simulink model "img2017"  (R2016b)
settings: Solver=VariableStepAuto  StartTime=0.0  StopTime=40  RelTol=1e-3
undefined symbols (not defined in the file or in its folder): none, Rec, SDTV, videoinput
libraries: visionanalysis x2, visiontransforms x2, dspmtrx3 x2, visionconversions x1, visiontextngfix x1, visionstatistics x1, imaqlib x1, visionsinks x1
settings Model: Creator=Anushri-MacBook  LastModifiedBy=Anushri-MacBook

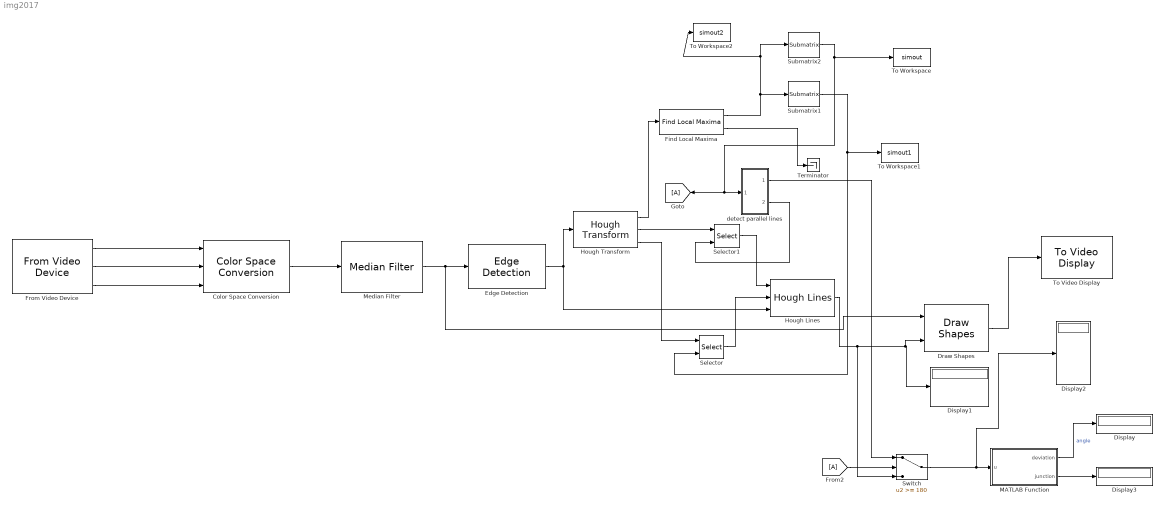
== system img2017 ==
  Color Space Conversion : visionconversions/Color Space  Conversion  conversion=Obsolete  conversionActive=R'G'B' to intensity  wp_str=D65  rec=Rec. 601 (SDTV)  sys=1125/60/2:1  imagePorts=Separate color signals
  Display{,1..3} (4 alike) : Display
  Draw Shapes : visiontextngfix/Draw Shapes  shape=Rectangles  fill=off  lineWidth=1  fillClrSource=Specify via dialog  display=Black  intensity=200  color=[0 255 0]  opacity=0.6  viewport=Entire image  antialiasing=off  inType=Obsolete  imagePorts=One multidimensional signal  prodOutputMode=Binary point scaling  prodOutputWordLength=32  prodOutputFracLength=14  memoryMode=Specify word length  memoryWordLength=16  memoryFracLength=15  roundingMode=Floor  overflowMode=off
  Edge Detection : visionanalysis/Edge Detection  method=Prewitt  outputType=Binary image  userDefinedThreshold=off  thresholdSource=Specify via dialog  threshold=0.1  thresholdTuning=8  edgeThinning=on  threshold_canny=[0.25 0.60]  autoPercent=40  sigma=1  prodOutputMode=Binary point scaling  prodOutputWordLength=32  prodOutputFracLength=8  roundingMode=Floor  overflowMode=off
  Find Local Maxima : visionstatistics/Find Local Maxima  num_peaks=2  nhood_size=[5 7]  src_thresh=Obsolete9b  src_thresh_inuse=Specify via dialog  threshold=10  inputIsHough=on  dt_peak=uint32  isOutVarDim=off  dt_count=uint32
  From Video Device : imaqlib/From Video Device  DeviceMenu=macvideo 1 (FaceTime HD Camera)  Device=macvideo 1 (USB2.0 PC CAMERA)  ObjConstructor=videoinput('macvideo', 1)  VideoFormatMenu=YCbCr422_1280x720  VideoFormat=YCbCr422_640x480  VideoSource=default  ROIPosition=[0 0 480 640]  EnableHWTrigger=off  TriggerConfiguration=none/none  SampleTime=1/30  OutputPortsMode=Separate color signals  DataType=single  CanDoHWTrigger=no  ReturnedColorSpace=rgb  BlockHandle=71.0071  ROIWidth=640  ROIHeight=480  ROIColumn=0  ROIRow=0  EngXMLPath=/Applications/MATLAB_R2016b.app/toolbox/imaq/imaq/private  DevXMLPath=/Users/Anushri-MacBook/Documents/MATLAB/SupportPackages/R2016b/toolbox/imaq/supportpackages/genericvideo/adaptor/maci64  EngLibPath=/Applications/MATLAB_R2016b.app/toolbox/imaq/imaqblks/imaqmex/maci64  ColorSpace=rgb  BayerSensorAlignment=grbg
  Hough Lines : visiontransforms/Hough Lines  sineCompMethod=Trigonometric function  thetaRes=pi/180  firstCoeffMode=Specify word length  firstCoeffWordLength=16  firstCoeffFracLength=15  prodOutputMode=Binary point scaling  prodOutputWordLength=32  prodOutputFracLength=16  roundingMode=Nearest  overflowMode=on
      settings: LockScale=on
  Hough Transform : visiontransforms/Hough Transform  theta_res=pi/180  rho_res=1  out_theta_rho=on  outdtmode=single  firstCoeffMode=Binary point scaling  firstCoeffWordLength=16  firstCoeffFracLength=14  secondCoeffMode=Binary point scaling  secondCoeffWordLength=32  secondCoeffFracLength=16  outputMode=Binary point scaling  outputWordLength=16  outputFracLength=0  accumMode=Binary point scaling  accumWordLength=32  accumFracLength=20  prodOutputMode=Binary point scaling  prodOutputWordLength=32  prodOutputFracLength=20  memoryMode=Binary point scaling  memoryWordLength=32  memoryFracLength=16  roundingMode=Nearest  overflowMode=on
  MATLAB Function : MATLAB Function  TreatAsAtomicUnit=on
  Median Filter : visionanalysis/Median Filter  nghbood=[2 2]  outSize=Same as input port I  padType=Symmetric  padSrc=Specify via dialog  padVal=0  roundingMode=Floor  overflowMode=off
  Selector : Selector  IndexMode=Zero-based  InputPortWidth=1599  IndexOptions=Index vector (port)  Indices=[1 3]  OutputSizes=1
  Selector1 : Selector  IndexMode=Zero-based  InputPortWidth=180  IndexOptions=Index vector (port)  Indices=[1 3]  OutputSizes=1
  Submatrix1 : dspmtrx3/Submatrix  RowSpan=One row  RowStartMode=Last  RowStartIndex=2  RowEndMode=Last  RowEndIndex=2937  ColSpan=One column  ColStartMode=Last  ColStartIndex=2  ColEndMode=Last  ColEndIndex=180
  Submatrix2 : dspmtrx3/Submatrix  RowSpan=One row  RowStartMode=First  RowStartIndex=1  RowEndMode=Middle  RowEndIndex=1  ColSpan=One column  ColStartMode=First  ColStartIndex=1  ColEndMode=Last  ColEndIndex=1
  Switch : Switch  Threshold=180
  Terminator : Terminator
  To Video Display : visionsinks/To Video Display  windowSizeMode=Normal  openAtMdlStart=on  fullScreen=off  videoWindowX=452  videoWindowY=130  saveWindowSize=off  videoWindowWidth=775  videoWindowHeight=508  inputColorFormat=RGB  inputType=Obsolete  imagePorts=One multidimensional signal  OutputDevice=On-screen video monitor  dataOrg=Column-major  isWindowOpen=off
  To Workspace : ToWorkspace  VariableName=simout  SaveFormat=Timeseries  SampleTime=-1
  To Workspace1 : ToWorkspace  VariableName=simout1  SaveFormat=Timeseries  SampleTime=-1
  To Workspace2 : ToWorkspace  VariableName=simout2  SaveFormat=Timeseries  SampleTime=-1
  detect parallel lines : Subsystem
  wires:
  From Video Device/1 -> Color Space Conversion/1
  From Video Device/2 -> Color Space Conversion/2
  From Video Device/3 -> Color Space Conversion/3
  Edge Detection/1 -> Hough Lines/3, Hough Transform/1
  Hough Transform/3 -> Selector/1
  Find Local Maxima/2 -> Terminator/1
  Hough Transform/1 -> Find Local Maxima/1
  Find Local Maxima/1 -> Submatrix1/1, To Workspace2/1, Submatrix2/1
  Selector/1 -> Hough Lines/2
  Selector1/1 -> Hough Lines/1
  Submatrix2/1 -> [A], detect parallel lines/1(In1), To Workspace/1
  Submatrix1/1 -> Selector/2, To Workspace1/1
  Median Filter/1 -> Draw Shapes/1, Edge Detection/1
  Draw Shapes/1 -> To Video Display/1
  MATLAB Function/1(deviation) -> Display/1  "angle"
  Color Space Conversion/1 -> Median Filter/1
  Hough Transform/2 -> Selector1/1
  detect parallel lines/2(Out2) -> Selector1/2
  Hough Lines/1 -> Draw Shapes/2, Display1/1, Switch/3
  Switch/1 -> Display2/1, MATLAB Function/1(u)
  [A] -> Switch/2
  detect parallel lines/1(Out1) -> Switch/1
  MATLAB Function/2(junction) -> Display3/1

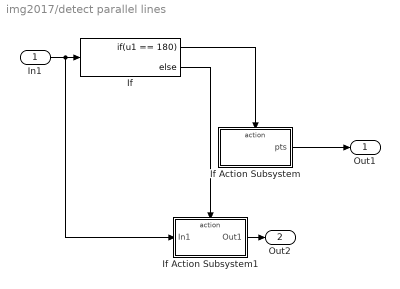
== system img2017/detect parallel lines ==
  In1 : Inport
  If : If  IfExpression=u1 == 180
  If Action Subsystem : Subsystem  TreatAsAtomicUnit=on
  If Action Subsystem1 : Subsystem  TreatAsAtomicUnit=on
  Out1 : Outport  OutDataTypeStr=int32
  Out2 : Outport  Port=2
  wires:
  If/2 -> If Action Subsystem1/Action
  In1/1 -> If Action Subsystem1/1(In1), If/1
  If Action Subsystem1/1(Out1) -> Out2/1
  If/1 -> If Action Subsystem/Action
  If Action Subsystem/1(pts) -> Out1/1

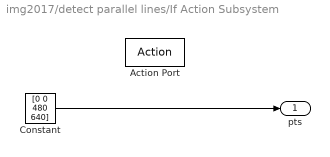
== system img2017/detect parallel lines/If Action Subsystem ==
  Action Port : ActionPort  ActionType=then
  Constant : Constant  Value=[0 0 480 640]  OutDataTypeStr=int32
  pts : Outport
  wires:
  Constant/1 -> pts/1

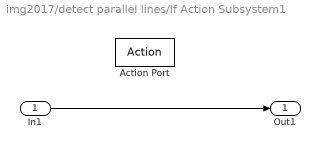
== system img2017/detect parallel lines/If Action Subsystem1 ==
  In1 : Inport
  Action Port : ActionPort  ActionType=else
  Out1 : Outport
  wires:
  In1/1 -> Out1/1

== matlab function img2017/MATLAB Function ==
  data: u input; deviation output; junction output
function [deviation,junction]= fcn(u)
%%initialize
xstart=u(1);
ystart=u(2);
xend=u(1)+u(3);
yend=u(2)+u(4);
n=480;
m=640;
%%calculate centre of rectangle drawn in image
xmid=xend-xstart;
ymid=yend-ystart;
centre_line=[xmid,ymid];
t1=double(centre_line);
%%deviation of rectangle centre from screen centre
OA=(t1-[n/2,m]);
OB=([n/2,m/2]-[n/2,m]);
deviation= anglevec(OA,OB);
junction = 0;
%%check for junction
if all(u==[0 0 0 0]) || all(u==[0 0 480 640])
    junction=1;
end
